simulink model "simplifiedSim"  (R2018b)
settings: Solver=VariableStepAuto  StartTime=0.0  StopTime=100  RelTol=1e-3
values from neighbouring files (symbols this model uses):
  GPS_time = [129600; 2034]    [simplifiedSim_init.m]
  t0 = simParams.time.epoch_utc_s    [simplifiedSim_init.m]
undefined symbols (not defined in the file or in its folder): clock_lib, DiscIntNeverNeededParam, Earth, fswParams, GPS_time_lib, magField_lib, satelliteDynamics_lib, sgp4, simParams, solarPressure_lib, time_coord_rotation_lib, WGS84
libraries: vrlib x4, aerolibutil x4, aerolibtransform2 x3, aerolibgravity2 x1, eclipseCheck x1, sunVector_lib x1, time_Lib x1, sgp4_lib_fsw x1, coord_rotation_lib x1, time_conversion_lib x1
settings Model: Creator=devantormey  LastModifiedBy=devantormey

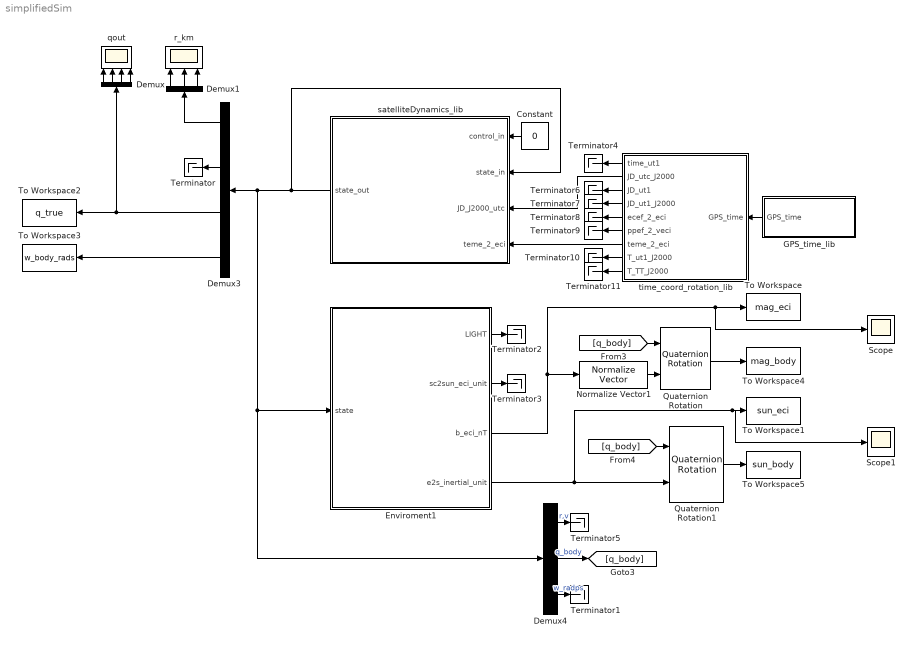
== system simplifiedSim ==
  Constant : Constant  Value=0
  Demux : Demux
  Demux1 : Demux  Outputs=3
  Demux3 : Demux  Outputs=[3 3 4 3]
  Demux4 : Demux  Outputs=[6 4 3]
  Enviroment1 : Subsystem
  GPS_time_lib : Subsystem  AncestorBlock=GPS_time_lib/GPS_time_lib
  Normalize Vector1 : vrlib/Utilities/Normalize Vector  maxzero=0
      settings: SourceProductName=Simulink 3D Animation  SourceProductBaseCode=VR
  Quaternion Rotation : aerolibutil/Quaternion Rotation
  Quaternion Rotation1 : aerolibutil/Quaternion Rotation
  Scope : Scope
  Scope1 : Scope
  Terminator{,1..11} (12 alike) : Terminator
  To Workspace : ToWorkspace  VariableName=mag_eci  SaveFormat=Timeseries  SampleTime=-1
  To Workspace1 : ToWorkspace  VariableName=sun_eci  SaveFormat=Timeseries  SampleTime=-1
  To Workspace2 : ToWorkspace  VariableName=q_true  SaveFormat=Timeseries  SampleTime=-1
  To Workspace3 : ToWorkspace  VariableName=w_body_rads  SaveFormat=Timeseries  SampleTime=-1
  To Workspace4 : ToWorkspace  VariableName=mag_body  SaveFormat=Timeseries  SampleTime=-1
  To Workspace5 : ToWorkspace  VariableName=sun_body  SaveFormat=Timeseries  SampleTime=-1
  qout : Scope  NumInputPorts=4
  r_km : Scope  NumInputPorts=3
  satelliteDynamics_lib : Subsystem  AncestorBlock=satelliteDynamics_lib/satelliteDynamics_lib
  time_coord_rotation_lib : Subsystem  AncestorBlock=time_coord_rotation_lib/time_coord_rotation_lib
  wires:
  Demux3/4 -> To Workspace3/1
  GPS_time_lib/1(GPS_time) -> time_coord_rotation_lib/1(GPS_time)
  Demux/4 -> qout/4
  Demux3/1 -> Demux1/1
  [q_body] -> Quaternion Rotation1/1
  Demux1/1 -> r_km/1
  Demux4/2 -> [q_body]  "q_body"
  Demux/3 -> qout/3
  time_coord_rotation_lib/2(JD_utc_J2000) -> satelliteDynamics_lib/3(JD_J2000_utc)
  [q_body] -> Quaternion Rotation/1
  Demux1/3 -> r_km/3
  Demux/1 -> qout/1
  Constant/1 -> satelliteDynamics_lib/1(control_in)
  Demux4/1 -> Terminator5/1  "r,v"
  satelliteDynamics_lib/1(state_out) -> satelliteDynamics_lib/2(state_in), Demux4/1, Enviroment1/1(state), Demux3/1
  Demux/2 -> qout/2
  time_coord_rotation_lib/7(teme_2_eci) -> satelliteDynamics_lib/4(teme_2_eci)
  Demux1/2 -> r_km/2
  Normalize Vector1/1 -> Quaternion Rotation/2
  Quaternion Rotation1/1 -> To Workspace5/1
  Demux3/3 -> Demux/1, To Workspace2/1
  Demux4/3 -> Terminator1/1  "w_radps"
  Quaternion Rotation/1 -> To Workspace4/1
  Demux3/2 -> Terminator/1
  Enviroment1/1(LIGHT) -> Terminator2/1
  Enviroment1/2(sc2sun_eci_unit) -> Terminator3/1
  time_coord_rotation_lib/1(time_ut1) -> Terminator4/1
  time_coord_rotation_lib/3(JD_ut1) -> Terminator6/1
  time_coord_rotation_lib/4(JD_ut1_J2000) -> Terminator7/1
  time_coord_rotation_lib/5(ecef_2_eci) -> Terminator8/1
  time_coord_rotation_lib/6(ppef_2_veci) -> Terminator9/1
  time_coord_rotation_lib/8(T_ut1_J2000) -> Terminator10/1
  time_coord_rotation_lib/9(T_TT_J2000) -> Terminator11/1
  Enviroment1/3(b_eci_nT) -> Scope/1, To Workspace/1, Normalize Vector1/1
  Enviroment1/4(e2s_inertial_unit) -> Scope1/1, To Workspace1/1, Quaternion Rotation1/2

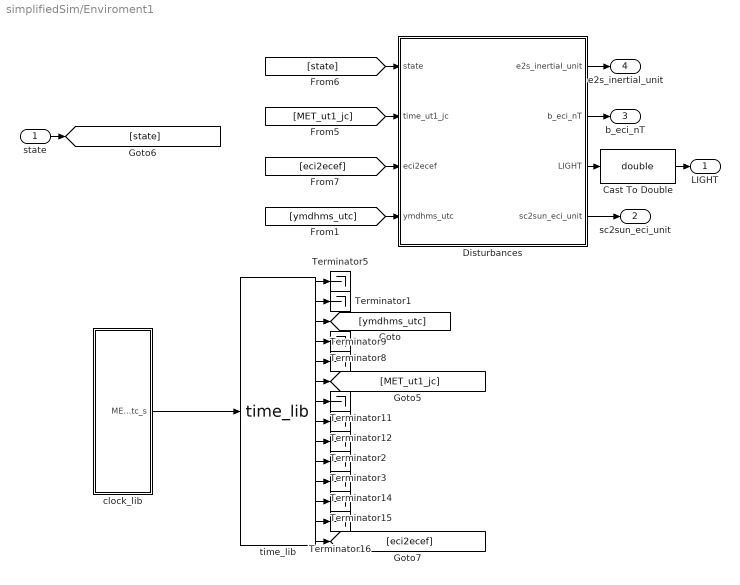
== system simplifiedSim/Enviroment1 ==
  state : Inport
  Cast To Double : DataTypeConversion  OutDataTypeStr=double
  Disturbances : Subsystem
  Terminator{1..3,5,8..9,11..12,14..16} (11 alike) : Terminator
  clock_lib : Subsystem  AncestorBlock=clock_lib/clock_lib
  "time_lib " : time_Lib/time_lib    SystemSampleTime=-1
  LIGHT : Outport
  sc2sun_eci_unit : Outport  Port=2
  b_eci_nT : Outport  Port=3
  e2s_inertial_unit : Outport  Port=4
  wires:
  state/1 -> [state]
  clock_lib/1(MET_utc_s) -> "time_lib "/1
  "time_lib "/14 -> [eci2ecef]
  [eci2ecef] -> Disturbances/3(eci2ecef)
  [MET_ut1_jc] -> Disturbances/2(time_ut1_jc)
  [state] -> Disturbances/1(state)
  Cast To Double/1 -> LIGHT/1
  Disturbances/3(LIGHT) -> Cast To Double/1
  "time_lib "/1 -> Terminator5/1
  "time_lib "/2 -> Terminator1/1
  "time_lib "/3 -> [ymdhms_utc]
  "time_lib "/4 -> Terminator8/1
  "time_lib "/5 -> Terminator9/1
  "time_lib "/6 -> [MET_ut1_jc]
  "time_lib "/7 -> Terminator11/1
  "time_lib "/8 -> Terminator12/1
  "time_lib "/9 -> Terminator2/1
  "time_lib "/11 -> Terminator14/1
  "time_lib "/12 -> Terminator15/1
  "time_lib "/13 -> Terminator16/1
  [ymdhms_utc] -> Disturbances/4(ymdhms_utc)
  Disturbances/4(sc2sun_eci_unit) -> sc2sun_eci_unit/1
  Disturbances/2(b_eci_nT) -> b_eci_nT/1
  Disturbances/1(e2s_inertial_unit) -> e2s_inertial_unit/1
  "time_lib "/10 -> Terminator3/1

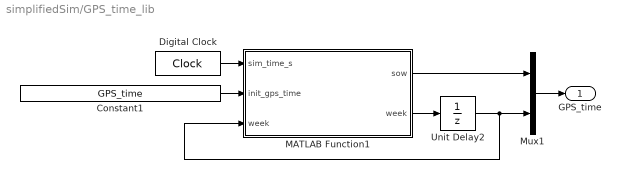
== system simplifiedSim/GPS_time_lib ==
  Constant1 : Constant  Value=GPS_time  VectorParams1D=off  SampleTime=-1
  Digital Clock : DigitalClock  SampleTime=.1
  MATLAB Function1 : MATLAB Function  TreatAsAtomicUnit=on
  Mux1 : Mux  Inputs=2
  Unit Delay2 : UnitDelay  InitialCondition=GPS_time(2)  SampleTime=-1
  GPS_time : Outport
  wires:
  Mux1/1 -> GPS_time/1
  MATLAB Function1/1(sow) -> Mux1/1
  Unit Delay2/1 -> Mux1/2, MATLAB Function1/3("week ")
  MATLAB Function1/2(week) -> Unit Delay2/1
  Constant1/1 -> MATLAB Function1/2(init_gps_time)
  Digital Clock/1 -> MATLAB Function1/1(sim_time_s)

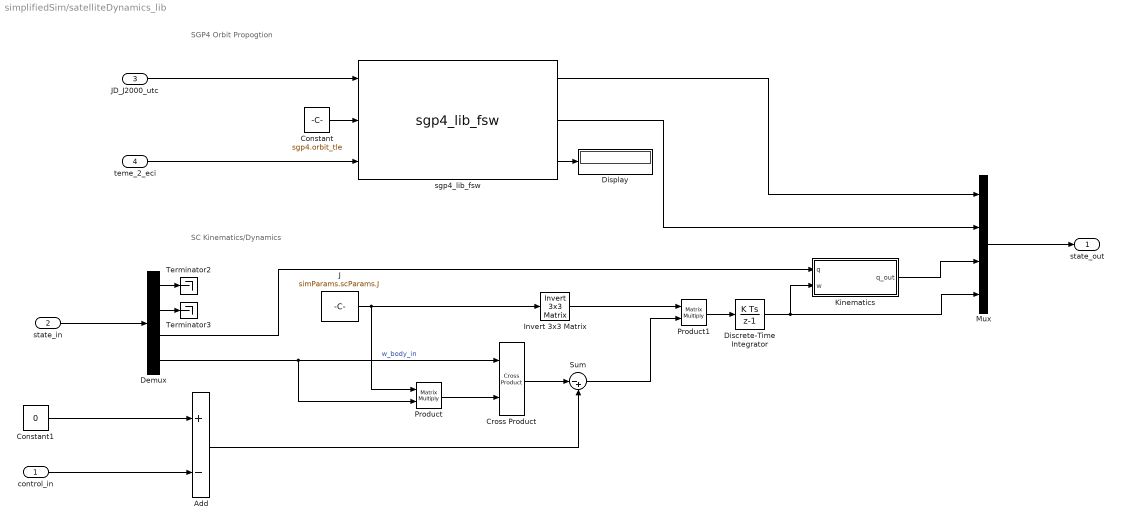
== system simplifiedSim/satelliteDynamics_lib ==
  note: SC Kinematics/Dynamics
  note: SGP4 Orbit Propogtion
  control_in : Inport
  state_in : Inport  Port=2
  JD_J2000_utc : Inport  Port=3
  teme_2_eci : Inport  Port=4
  Add : Sum  Inputs=+-
  Constant : Constant  Value=sgp4.orbit_tle
  Constant1 : Constant  Value=0
  Cross Product : vrlib/Utilities/Cross Product
      settings: SourceProductBaseCode=VR
  Demux : Demux  Outputs=[3 3 4 3]
  Discrete-Time Integrator : DiscreteIntegrator  InitialCondition=simParams.initialConditions.w0  SampleTime=-1  ICPrevOutput=DiscIntNeverNeededParam  ICPrevScaledInput=DiscIntNeverNeededParam
  Display : Display
  Invert 3x3 Matrix : aerolibutil/Invert  3x3 Matrix
  J : Constant  Value=simParams.scParams.J
  Kinematics : Subsystem
  Mux : Mux  Inputs=[3 3 4 3]
  Product : Product  Multiplication=Matrix(*)
  Product1 : Product  Multiplication=Matrix(*)
  Sum : Sum  Inputs=|-+
  Terminator2 : Terminator
  Terminator3 : Terminator
  sgp4_lib_fsw : sgp4_lib_fsw/sgp4_lib_fsw  SystemSampleTime=-1
  state_out : Outport
  wires:
  Demux/2 -> Terminator3/1
  Add/1 -> Sum/2
  control_in/1 -> Add/2
  Constant1/1 -> Add/1
  state_in/1 -> Demux/1
  Mux/1 -> state_out/1
  Demux/1 -> Terminator2/1
  Demux/3 -> Kinematics/1(q)
  Demux/4 -> Product/2, Cross Product/1  "w_body_in"
  Kinematics/1(q_out) -> Mux/3
  Discrete-Time Integrator/1 -> Kinematics/2(w), Mux/4
  Product1/1 -> Discrete-Time Integrator/1
  Invert 3x3 Matrix/1 -> Product1/1
  Sum/1 -> Product1/2
  Cross Product/1 -> Sum/1
  Product/1 -> Cross Product/2
  J/1 -> Invert 3x3 Matrix/1, Product/1
  sgp4_lib_fsw/1 -> Mux/1
  sgp4_lib_fsw/2 -> Mux/2
  sgp4_lib_fsw/3 -> Display/1
  Constant/1 -> sgp4_lib_fsw/2
  teme_2_eci/1 -> sgp4_lib_fsw/3
  JD_J2000_utc/1 -> sgp4_lib_fsw/1

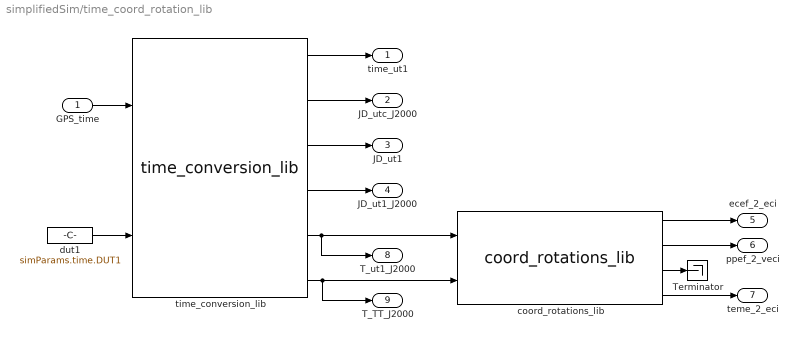
== system simplifiedSim/time_coord_rotation_lib ==
  GPS_time : Inport
  Terminator : Terminator
  coord_rotations_lib : coord_rotation_lib/coord_rotations_lib  SystemSampleTime=-1
  dut1 : Constant  Value=simParams.time.DUT1
  time_conversion_lib : time_conversion_lib/time_conversion_lib  SystemSampleTime=-1
  time_ut1 : Outport
  JD_utc_J2000 : Outport  Port=2
  JD_ut1 : Outport  Port=3
  JD_ut1_J2000 : Outport  Port=4
  ecef_2_eci : Outport  Port=5
  ppef_2_veci : Outport  Port=6
  teme_2_eci : Outport  Port=7
  T_ut1_J2000 : Outport  Port=8
  T_TT_J2000 : Outport  Port=9
  wires:
  dut1/1 -> time_conversion_lib/2
  time_conversion_lib/5 -> T_ut1_J2000/1, coord_rotations_lib/1
  time_conversion_lib/6 -> T_TT_J2000/1, coord_rotations_lib/2
  time_conversion_lib/1 -> time_ut1/1
  time_conversion_lib/3 -> JD_ut1/1
  time_conversion_lib/4 -> JD_ut1_J2000/1
  coord_rotations_lib/1 -> ecef_2_eci/1
  coord_rotations_lib/2 -> ppef_2_veci/1
  coord_rotations_lib/4 -> teme_2_eci/1
  coord_rotations_lib/3 -> Terminator/1
  time_conversion_lib/2 -> JD_utc_J2000/1
  GPS_time/1 -> time_conversion_lib/1

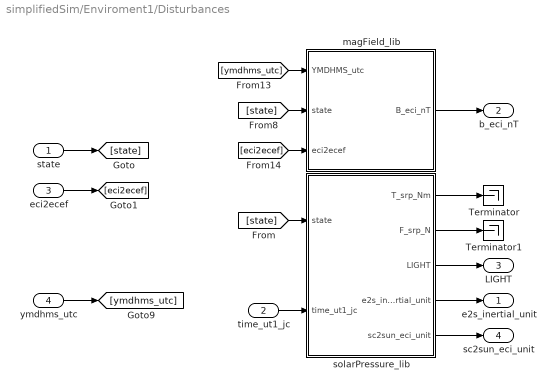
== system simplifiedSim/Enviroment1/Disturbances ==
  state : Inport
  time_ut1_jc : Inport  Port=2
  eci2ecef : Inport  Port=3
  ymdhms_utc : Inport  Port=4
  Terminator : Terminator
  Terminator1 : Terminator
  magField_lib : Subsystem  AncestorBlock=magField_lib/magField_lib
  solarPressure_lib : Subsystem  AncestorBlock=solarPressure_lib/solarPressure_lib
  e2s_inertial_unit : Outport
  b_eci_nT : Outport  Port=2
  LIGHT : Outport  Port=3
  sc2sun_eci_unit : Outport  Port=4
  wires:
  solarPressure_lib/3(LIGHT) -> LIGHT/1
  solarPressure_lib/1(T_srp_Nm) -> Terminator/1
  solarPressure_lib/4(e2s_inertial_unit) -> e2s_inertial_unit/1
  solarPressure_lib/2(F_srp_N) -> Terminator1/1
  time_ut1_jc/1 -> solarPressure_lib/2(time_ut1_jc)
  state/1 -> [state]
  [state] -> solarPressure_lib/1(state)
  eci2ecef/1 -> [eci2ecef]
  [state] -> magField_lib/2(state)
  ymdhms_utc/1 -> [ymdhms_utc]
  [ymdhms_utc] -> magField_lib/1(YMDHMS_utc)
  [eci2ecef] -> magField_lib/3(eci2ecef)
  magField_lib/1(B_eci_nT) -> b_eci_nT/1
  solarPressure_lib/5(sc2sun_eci_unit) -> sc2sun_eci_unit/1

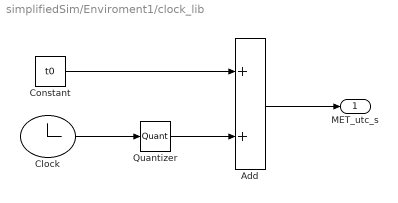
== system simplifiedSim/Enviroment1/clock_lib ==
  Add : Sum
  Clock : Clock
  Constant : Constant  Value=t0
  Quantizer : Quantizer  QuantizationInterval=simParams.time.res
  MET_utc_s : Outport
  wires:
  Add/1 -> MET_utc_s/1
  Quantizer/1 -> Add/2
  Constant/1 -> Add/1
  Clock/1 -> Quantizer/1

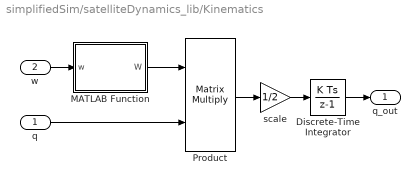
== system simplifiedSim/satelliteDynamics_lib/Kinematics ==
  q : Inport
  w : Inport  Port=2
  Discrete-Time Integrator : DiscreteIntegrator  InitialCondition=simParams.initialConditions.q0  SampleTime=-1  ICPrevOutput=DiscIntNeverNeededParam  ICPrevScaledInput=DiscIntNeverNeededParam
  MATLAB Function : MATLAB Function  TreatAsAtomicUnit=on
  Product : Product  Multiplication=Matrix(*)
  scale : Gain  Gain=1/2
  q_out : Outport
  wires:
  Discrete-Time Integrator/1 -> q_out/1
  scale/1 -> Discrete-Time Integrator/1
  Product/1 -> scale/1
  q/1 -> Product/2
  MATLAB Function/1(W) -> Product/1
  w/1 -> MATLAB Function/1(w)

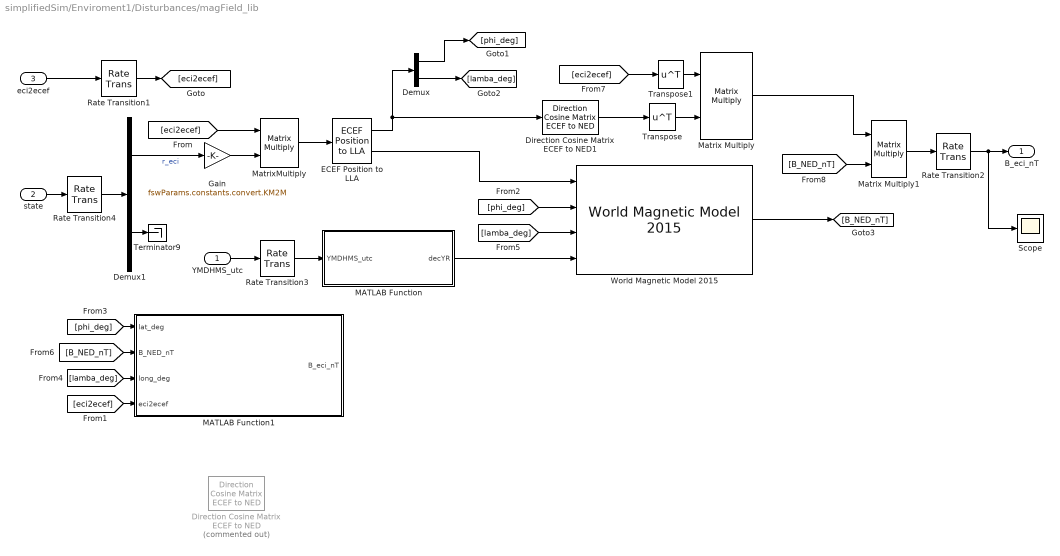
== system simplifiedSim/Enviroment1/Disturbances/magField_lib ==
  YMDHMS_utc : Inport
  state : Inport  Port=2
  eci2ecef : Inport  Port=3
  Demux : Demux  Outputs=[1 1]
  Demux1 : Demux  Outputs=[3 10]
  Direction Cosine Matrix ECEF to NED : aerolibtransform2/Direction Cosine Matrix ECEF to NED  Commented=on
      settings: SourceProductName=Aerospace Blockset  SourceProductBaseCode=AE
  Direction Cosine Matrix ECEF to NED1 : aerolibtransform2/Direction Cosine Matrix ECEF to NED
      settings: SourceProductName=Aerospace Blockset  SourceProductBaseCode=AE
  ECEF Position to LLA : aerolibtransform2/ECEF Position to LLA  units=Metric (MKS)  ptype=Earth (WGS84)  F=1/298.257223563  R=6378137
      settings: SourceProductName=Aerospace Blockset  SourceProductBaseCode=AE
  Gain : Gain  Gain=fswParams.constants.convert.KM2M
  MATLAB Function : MATLAB Function  TreatAsAtomicUnit=on
  MATLAB Function1 : MATLAB Function  TreatAsAtomicUnit=on
  Matrix Multiply : Product  Multiplication=Matrix(*)
  Matrix Multiply1 : Product  Multiplication=Matrix(*)
  MatrixMultiply : Product  Multiplication=Matrix(*)
  Rate Transition1 : RateTransition  OutPortSampleTime=simParams.magField.sample_time_s
  Rate Transition2 : RateTransition
  Rate Transition3 : RateTransition  OutPortSampleTime=simParams.magField.sample_time_s
  Rate Transition4 : RateTransition  OutPortSampleTime=simParams.magField.sample_time_s
  Scope : Scope
  Terminator9 : Terminator
  Transpose : Math  Operator=transpose  SaturateOnIntegerOverflow=on
  Transpose1 : Math  Operator=transpose  SaturateOnIntegerOverflow=on
  World Magnetic Model 2015 : aerolibgravity2/World Magnetic Model 2015  units=Metric (MKS)  time_in=on  month=January  day=1  year=2015  action=Error  h_out=off  dec_out=off  inc_out=off  ti_out=off
      settings: SourceProductName=Aerospace Blockset  SourceProductBaseCode=AE
  B_eci_nT : Outport
  wires:
  [lamba_deg] -> MATLAB Function1/3(long_deg)
  [B_NED_nT] -> MATLAB Function1/2(B_NED_nT)
  World Magnetic Model 2015/1 -> [B_NED_nT]
  [lamba_deg] -> World Magnetic Model 2015/3
  [phi_deg] -> MATLAB Function1/1(lat_deg)
  [phi_deg] -> World Magnetic Model 2015/2
  Rate Transition3/1 -> MATLAB Function/1(YMDHMS_utc)
  Rate Transition1/1 -> [eci2ecef]
  Rate Transition4/1 -> Demux1/1
  [eci2ecef] -> MATLAB Function1/4(eci2ecef)
  [eci2ecef] -> MatrixMultiply/1
  eci2ecef/1 -> Rate Transition1/1
  state/1 -> Rate Transition4/1
  Demux1/1 -> Gain/1  "r_eci"
  Demux1/2 -> Terminator9/1
  YMDHMS_utc/1 -> Rate Transition3/1
  MATLAB Function/1(decYR) -> World Magnetic Model 2015/4
  MatrixMultiply/1 -> ECEF Position to LLA/1
  ECEF Position to LLA/2 -> World Magnetic Model 2015/1
  ECEF Position to LLA/1 -> Direction Cosine Matrix ECEF to NED1/1, Demux/1
  Demux/1 -> [phi_deg]
  Demux/2 -> [lamba_deg]
  Direction Cosine Matrix ECEF to NED1/1 -> Transpose/1
  [eci2ecef] -> Transpose1/1
  Transpose1/1 -> Matrix Multiply/1
  Transpose/1 -> Matrix Multiply/2
  Matrix Multiply/1 -> Matrix Multiply1/1
  [B_NED_nT] -> Matrix Multiply1/2
  Rate Transition2/1 -> Scope/1, B_eci_nT/1
  Matrix Multiply1/1 -> Rate Transition2/1
  Gain/1 -> MatrixMultiply/2

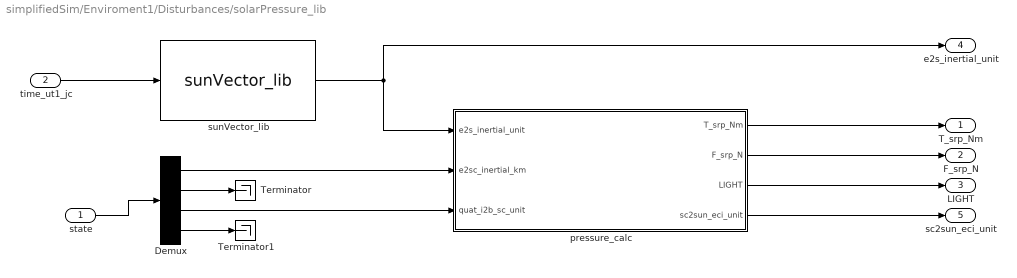
== system simplifiedSim/Enviroment1/Disturbances/solarPressure_lib ==
  state : Inport
  time_ut1_jc : Inport  Port=2
  Demux : Demux  Outputs=[3 3 4 3]
  Terminator : Terminator
  Terminator1 : Terminator
  pressure_calc : Subsystem
  sunVector_lib : sunVector_lib/sunVector_lib  SystemSampleTime=-1
  T_srp_Nm : Outport
  F_srp_N : Outport  Port=2
  LIGHT : Outport  Port=3
  e2s_inertial_unit : Outport  Port=4
  sc2sun_eci_unit : Outport  Port=5
  wires:
  pressure_calc/3(LIGHT) -> LIGHT/1
  state/1 -> Demux/1
  Demux/4 -> Terminator1/1
  time_ut1_jc/1 -> sunVector_lib/1
  Demux/1 -> pressure_calc/2(e2sc_inertial_km)
  Demux/2 -> Terminator/1
  Demux/3 -> pressure_calc/3(quat_i2b_sc_unit)
  pressure_calc/1(T_srp_Nm) -> T_srp_Nm/1
  sunVector_lib/1 -> e2s_inertial_unit/1, pressure_calc/1(e2s_inertial_unit)
  pressure_calc/2(F_srp_N) -> F_srp_N/1
  pressure_calc/4(sc2sun_eci_unit) -> sc2sun_eci_unit/1

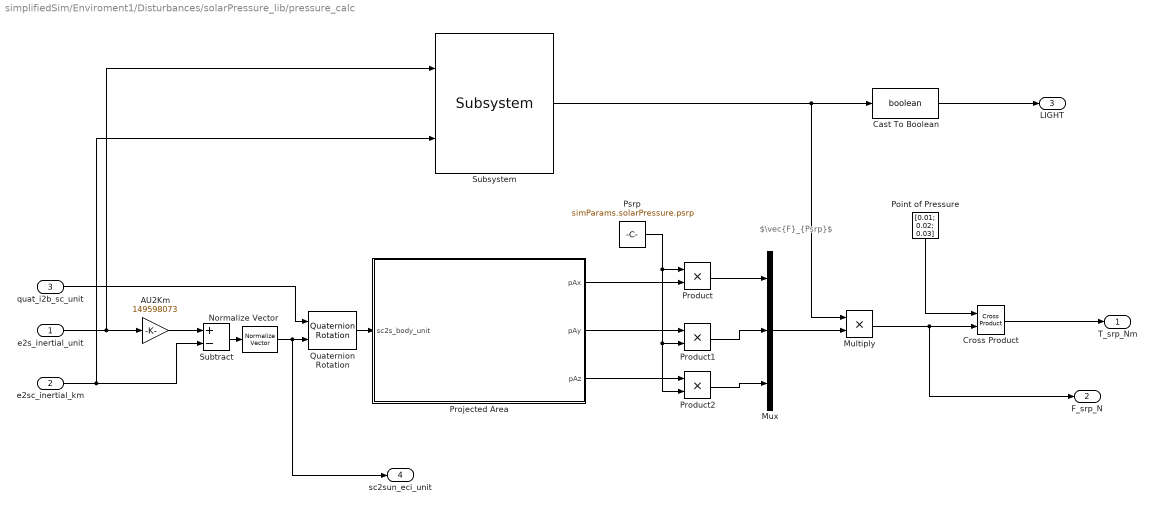
== system simplifiedSim/Enviroment1/Disturbances/solarPressure_lib/pressure_calc ==
  note: $\vec{F}_{Psrp}$
  e2s_inertial_unit : Inport
  e2sc_inertial_km : Inport  Port=2
  quat_i2b_sc_unit : Inport  Port=3
  AU2Km : Gain  Gain=149598073
  Cast To Boolean : DataTypeConversion  OutDataTypeStr=boolean
  Cross Product : vrlib/Utilities/Cross Product
      settings: SourceProductBaseCode=VR
  Multiply : Product
  Mux : Mux  Inputs=3
  Normalize Vector : vrlib/Utilities/Normalize Vector  maxzero=0
      settings: SourceProductName=Simulink 3D Animation  SourceProductBaseCode=VR
  Point of Pressure : Constant  Value=[0.01; 0.02; 0.03]
  Product : Product
  Product1 : Product
  Product2 : Product
  Projected Area : Subsystem
  Psrp : Constant  Value=simParams.solarPressure.psrp
  Quaternion Rotation : aerolibutil/Quaternion Rotation
  Subsystem : eclipseCheck/Subsystem  SystemSampleTime=-1
  Subtract : Sum  Inputs=+-
  T_srp_Nm : Outport
  F_srp_N : Outport  Port=2
  LIGHT : Outport  Port=3
  sc2sun_eci_unit : Outport  Port=4
  wires:
  Normalize Vector/1 -> sc2sun_eci_unit/1, Quaternion Rotation/2
  Subtract/1 -> Normalize Vector/1
  AU2Km/1 -> Subtract/1
  Cast To Boolean/1 -> LIGHT/1
  Subsystem/1 -> Multiply/1, Cast To Boolean/1
  Multiply/1 -> Cross Product/2, F_srp_N/1
  Mux/1 -> Multiply/2
  Quaternion Rotation/1 -> Projected Area/1(sc2s_body_unit)
  quat_i2b_sc_unit/1 -> Quaternion Rotation/1
  e2sc_inertial_km/1 -> Subsystem/2, Subtract/2
  e2s_inertial_unit/1 -> Subsystem/1, AU2Km/1
  Cross Product/1 -> T_srp_Nm/1
  Point of Pressure/1 -> Cross Product/1
  Product2/1 -> Mux/3
  Product1/1 -> Mux/2
  Product/1 -> Mux/1
  Projected Area/3(pAz) -> Product2/1
  Projected Area/2(pAy) -> Product1/1
  Psrp/1 -> Product/1, Product1/2, Product2/2
  Projected Area/1(pAx) -> Product/2

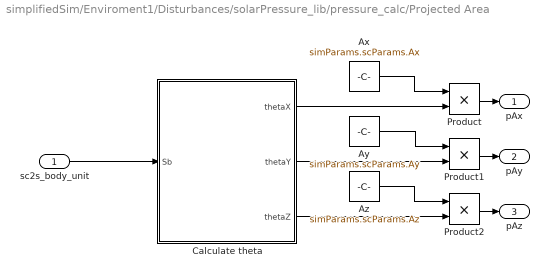
== system simplifiedSim/Enviroment1/Disturbances/solarPressure_lib/pressure_calc/Projected Area ==
  sc2s_body_unit : Inport
  Ax : Constant  Value=simParams.scParams.Ax
  Ay : Constant  Value=simParams.scParams.Ay
  Az : Constant  Value=simParams.scParams.Az
  Calculate theta : MATLAB Function  TreatAsAtomicUnit=on
  Product : Product
  Product1 : Product
  Product2 : Product
  pAx : Outport
  pAy : Outport  Port=2
  pAz : Outport  Port=3
  wires:
  Ax/1 -> Product/1
  sc2s_body_unit/1 -> Calculate theta/1(Sb)
  Product/1 -> pAx/1
  Calculate theta/2(thetaY) -> Product1/2
  Calculate theta/1(thetaX) -> Product/2
  Ay/1 -> Product1/1
  Calculate theta/3(thetaZ) -> Product2/2
  Az/1 -> Product2/1
  Product2/1 -> pAz/1
  Product1/1 -> pAy/1

== matlab function simplifiedSim/Enviroment1/Disturbances/magField_lib/MATLAB Function ==
  data: YMDHMS_utc input; decYR output
%function converts YMDHMS array to decimal years
function decYR = decyr(YMDHMS_utc)
year=YMDHMS_utc(1);
month=YMDHMS_utc(2);
day=YMDHMS_utc(3);
hour=YMDHMS_utc(4);
min=YMDHMS_utc(5);
sec=YMDHMS_utc(6);

janD=31;
marchD=31;
aprilD=30;
mayD=31;
juneD=30;
julyD=31; 
augD=31;
septD=30;
octD=31;
novD=30;



if mod(year,4)==0 %leap year
    daysT=366; %total days in year
    fedD=29;
else
    daysT=365.25;
    fedD=28;
end
    
if month == 1
    daysS= day; %days so far
elseif month ==2
    daysS=janD+day;
elseif month ==3
    daysS=janD+fedD+day;
elseif month==4
    daysS=janD+fedD+marchD+day;
elseif month==5
    daysS=janD+fedD+marchD+aprilD+day;
elseif month==6
    daysS=janD+fedD+marchD+aprilD+mayD+day;
elseif month==7
    daysS=janD+fedD+marchD+aprilD+mayD+juneD+day;
elseif month==8
    daysS=janD+fedD+marchD+aprilD+mayD+juneD+julyD+day;
elseif month==9
    daysS=janD+fedD+marchD+aprilD+mayD+juneD+julyD+augD+day;
elseif month==10
    daysS=janD+fedD+marchD+aprilD+mayD+juneD+julyD+augD+septD+day;
elseif month==11
    daysS=janD+fedD+marchD+aprilD+mayD+juneD+julyD+augD+septD+octD+day;
else %dec
    daysS=janD+fedD+marchD+aprilD+mayD+juneD+julyD+augD+septD+octD+novD+day;
end

%add time of day component
daysS=daysS+hour/24+min/1440+sec/86400;
decYR=year+daysS/daysT;
end

== matlab function simplifiedSim/satelliteDynamics_lib/Kinematics/MATLAB Function ==
  data: w input; W output
function W = fcn(w)
%#codegen

W = [0, -w(1),-w(2),-w(3); w(1), 0,w(3), -w(2); w(2), -w(3), 0, w(1); w(3), w(2), -w(1), 0 ];

end

== matlab function simplifiedSim/GPS_time_lib/MATLAB Function1 ==
  data: sim_time_s input; sow output; init_gps_time input; week input; week output
function [sow, week] = gps_clock(sim_time_s, init_gps_time, week)
% ----------------------------------------------------------------------- %
% UW HuskySat-1, ADCS Subsystem
%
% GPS clock for the SIM.
% ----------------------------------------------------------------------- %

% Constants
sec_in_week = 604800;


init_sow    = init_gps_time(1);
sow         = mod(init_sow + sim_time_s, sec_in_week);

% Handle roll overs
if sow == sec_in_week
    week = week + 1;
end

end

== matlab function simplifiedSim/Enviroment1/Disturbances/solarPressure_lib/pressure_calc/Projected Area/Calculate theta ==
  data: Sb input; thetaX output; thetaY output; thetaZ output
% Author: Devan Tormey
% Date: 2/21/2019
function [thetaX,thetaY,thetaZ] = fcn(Sb)
% Description: This function computes the dot product of the sun vector
% with the appropriate body coordinate vector.
%~~~~~~~~~~~~~ 
%  Variables 
%~~~~~~~~~~~~~~
% Sb - this is the sun vector (calculated elsewhere)
% ThetaXYZ - as these are all unit vectors the dot product produces the
% cosine of the angle in between

    if Sb(1) >= 0 
        thetaX = dot(Sb,[1;0;0]);
    else 
        thetaX = dot(Sb,[-1;0;0]);
    end

    if Sb(2) >= 0 
        thetaY = dot(Sb,[0;1;0]);
    else 
        thetaY = dot(Sb,[0;-1;0]);
    end

    if Sb(3) >= 0 
        thetaZ = dot(Sb,[0;0;1]);
    else 
        thetaZ = dot(Sb,[0;0;-1]);
    end

end

== matlab function simplifiedSim/Enviroment1/Disturbances/magField_lib/MATLAB Function1 ==
  data: lat_deg input; B_NED_nT input; B_eci_nT output; long_deg input; eci2ecef input
function B_eci_nT = ned2eci(lat_deg,B_NED_nT,long_deg,eci2ecef)
%NED to ECEF
DCMef=zeros(3);
%source:https://www.mathworks.com/help/aeroblks/directioncosinematrixeceftoned.html
DCMef=[-sind(lat_deg)*cosd(long_deg) -sind(lat_deg)*sind(long_deg) cosd(lat_deg);...
    -sind(long_deg) cosd(long_deg) 0;...
    -cosd(lat_deg)*cosd(long_deg) -cosd(lat_deg)*sind(long_deg) -sind(lat_deg)];

B_ecef=transpose(DCMef)*B_NED_nT;

%ECEF to ECI using transformation matrix from time lib
B_eci_nT=transpose(eci2ecef)*B_ecef; %eci2ecef transformation matrix given by time_lib
end
